simulink model "real_LAB3_SS"  (R2025b)
settings: Solver=ode3  StartTime=0.0  StopTime=10  FixedStep=0.001  RelTol=1e-3
values from neighbouring files (symbols this model uses):
  deltac = 1/sqrt(2)    [real_LAB3.m]    (also in sim_LAB3.m)
  K = lqr(sysG,Q,R)    [diScorta.m]    (also in real_LAB3.m; sim_LAB3.m = place(A, B,lamb))
  Nu = N(5)    [diScorta.m]    (also in real_LAB3.m; sim_LAB3.m)
  Nx = N(1:4)    [diScorta.m]    (also in real_LAB3.m; sim_LAB3.m)
  step_amplitude = 50    [diScorta.m]    (also in real_LAB3.m)
  t0 = 0.2    [diScorta.m]    (also in real_LAB3.m; real_estimation.m)
  t1 = 0.7    [diScorta.m]    (also in real_LAB3.m; real_estimation.m)
  Ts = 0.001    [diScorta.m]    (also in real_LAB3.m; real_estimation.m; sim_LAB3.m)
  wc = 2*pi*50    (= 314.159265359)    [real_LAB3.m]    (also in sim_LAB3.m)
undefined symbols (not defined in the file or in its folder): degs2rpm, DiscIntNeverNeededParam, National_Instruments, PCI, rpm2rads, sens
libraries: sldrtlib x3, simulink x1
settings Model: SimulationMode=external  ExtModeTrigDuration=100001  Creator=delpratogi  LastModifiedBy=ester
settings DataIOCC: ReturnWorkspaceOutputs=off
settings HardwareCC: ProdBitPerLong=64.0  ProdHWDeviceType=Intel->x86-64 (Linux 64)
settings RTWCC: SystemTargetFile=sldrt.tlc  TemplateMakefile=sldrt.tmf  RTWCompilerOptimization=on  Description=Simulink Desktop Real-Time
settings CodeAppCC: MaxIdLength=95.0
settings SimulinkDesktopRealTimeCC: ExtModeTransport=0.0  ExtModeStaticAllocSize=1000000.0  TargetLibSuffix=_sldrt.a  TargetPreCompLibLocation=C:\Program Files\MATLAB\R2025b\toolbox\sldrt\lib\win64  MultiwordLength=2048.0  DynamicStringBufferSize=256.0  ParMdlRefBuildCompliant=on  PreserveMATLABNamespacesInGeneratedCode=on  SubcomponentCodeInterfacePackaging=Reusable function

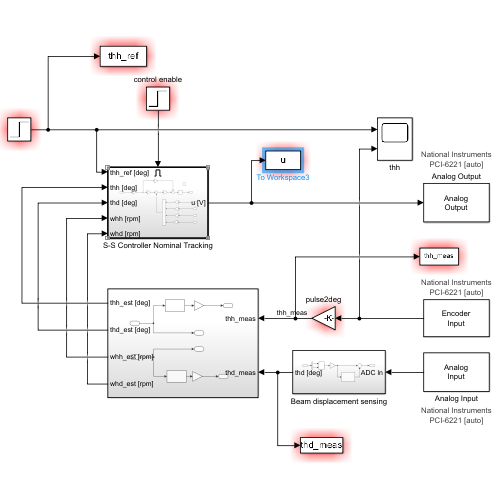
[thumbnail: Simulink's stored preview of the top-level diagram]
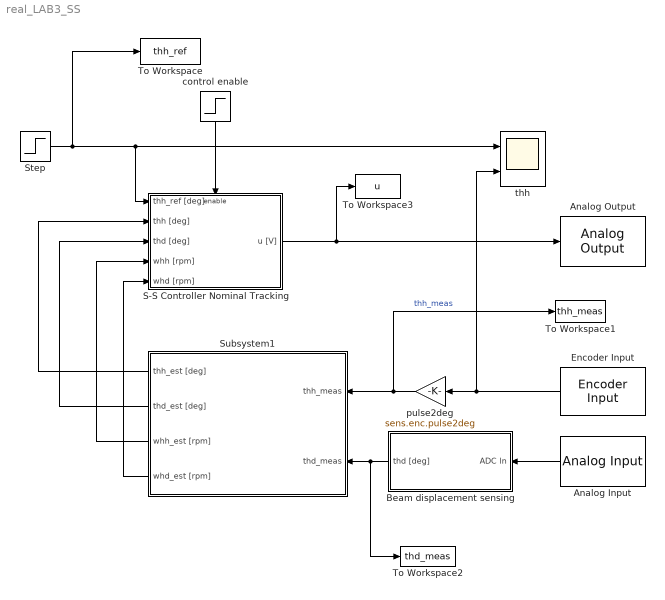
== system real_LAB3_SS ==
  Analog Input : sldrtlib/Analog Input  SampleTime=0.001  MaxMissedTicks=10  ShowMissedTicks=off  YieldWhenWaiting=off  DrvName=National_Instruments/PCI-6221  DrvAddress=4294967295  DrvOptions=[0 0 0 2 0]  Channels=[3,2]  RangeMode=1  VoltRange=2  DataType=1
      settings: AttributesFormatString=National Instruments\nPCI-6221 [auto]
  Analog Output : sldrtlib/Analog Output  SampleTime=0.001  MaxMissedTicks=10  ShowMissedTicks=off  YieldWhenWaiting=off  DrvName=National_Instruments/PCI-6221  DrvAddress=4294967295  DrvOptions=[0 0 0 2 0]  Channels=1  RangeMode=1  VoltRange=1  InitialValue=0  FinalValue=0
      settings: AttributesFormatString=National Instruments\nPCI-6221 [auto]
  Beam displacement sensing : Subsystem
  Encoder Input : sldrtlib/Encoder Input  SampleTime=0.001  MaxMissedTicks=10  ShowMissedTicks=off  YieldWhenWaiting=off  DrvName=National_Instruments/PCI-6221  DrvAddress=4294967295  DrvOptions=[0 0 0 2 0]  Channels=1  QuadMode=3  IndexPulse=1  InputFilter=Inf  DataType=1
      settings: AttributesFormatString=National Instruments\nPCI-6221 [auto]
  S-S Controller Nominal Tracking : Subsystem
  Step : Step  After=step_amplitude  SampleTime=Ts
  Subsystem1 : Subsystem
  To Workspace : ToWorkspace  VariableName=thh_ref  SaveFormat=Structure With Time  SampleTime=Ts
  To Workspace1 : ToWorkspace  VariableName=thh_meas  SaveFormat=Structure With Time  SampleTime=Ts
  To Workspace2 : ToWorkspace  VariableName=thd_meas  SaveFormat=Structure With Time  SampleTime=Ts
  To Workspace3 : ToWorkspace  VariableName=u  SaveFormat=Structure With Time  SampleTime=Ts
  control enable : Step  Time=t1  SampleTime=0
  pulse2deg : Gain  Gain=sens.enc.pulse2deg
  thh : Scope  NumInputPorts=2
      settings: ActiveDisplayYMinimum=-6.2503462089638822  ActiveDisplayYMaximum=56.250038467662655
  wires:
  Analog Input/1 -> Beam displacement sensing/1(ADC ln)
  Subsystem1/2(thd_est [deg]) -> S-S Controller Nominal Tracking/3(thd [deg])
  Step/1 -> To Workspace/1, S-S Controller Nominal Tracking/1(thh_ref [deg]), thh/1
  Subsystem1/3(whh_est [rpm]) -> S-S Controller Nominal Tracking/4(whh [rpm])
  S-S Controller Nominal Tracking/1(u [V]) -> To Workspace3/1, Analog Output/1
  Encoder Input/1 -> thh/2, pulse2deg/1
  Subsystem1/1(thh_est [deg]) -> S-S Controller Nominal Tracking/2(thh [deg])
  Subsystem1/4(whd_est [rpm]) -> S-S Controller Nominal Tracking/5(whd [rpm])
  pulse2deg/1 -> To Workspace1/1, Subsystem1/1(thh_meas)  "thh_meas"
  Beam displacement sensing/1(thd [deg]) -> To Workspace2/1, Subsystem1/2(thd_meas)
  control enable/1 -> S-S Controller Nominal Tracking/Enable

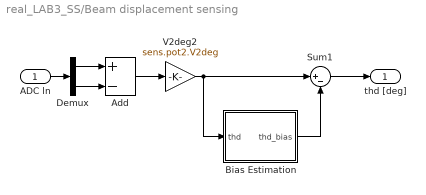
== system real_LAB3_SS/Beam displacement sensing ==
  ADC ln : Inport
  Add : Sum  Inputs=+-
  Bias Estimation : Subsystem
  Demux : Demux  Outputs=2
  Sum1 : Sum  Inputs=|+-
  V2deg2 : Gain  Gain=sens.pot2.V2deg
  thd [deg] : Outport
  wires:
  V2deg2/1 -> Sum1/1, Bias Estimation/1(thd)
  Sum1/1 -> thd [deg]/1
  Bias Estimation/1(thd_bias) -> Sum1/2
  Add/1 -> V2deg2/1
  Demux/1 -> Add/1
  ADC ln/1 -> Demux/1
  Demux/2 -> Add/2

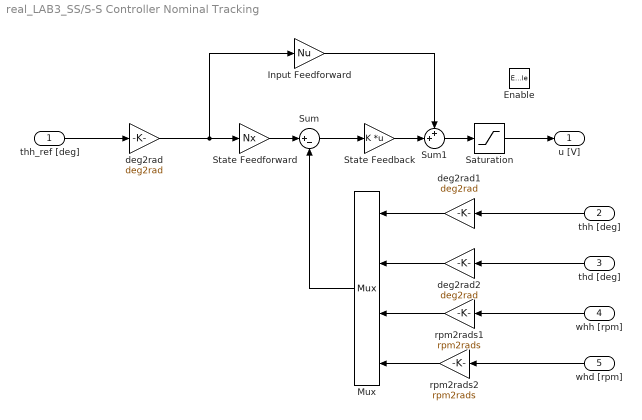
== system real_LAB3_SS/S-S Controller Nominal Tracking ==
  thh_ref [deg] : Inport
  thh [deg] : Inport  Port=2
  thd [deg] : Inport  Port=3
  whh [rpm] : Inport  Port=4
  whd [rpm] : Inport  Port=5
  Enable : EnablePort
  Input Feedforward : Gain  Gain=Nu
  Mux : Mux
  Saturation : Saturate  UpperLimit=10  LowerLimit=-10  ZeroCross=off
  State Feedback : Gain  Gain=K  Multiplication=Matrix(K*u)
  State Feedforward : Gain  Gain=Nx
  Sum : Sum  Inputs=|+-
  Sum1 : Sum  Inputs=++|
  deg2rad : Gain  Gain=deg2rad
  deg2rad1 : Gain  Gain=deg2rad
  deg2rad2 : Gain  Gain=deg2rad
  rpm2rads1 : Gain  Gain=rpm2rads
  rpm2rads2 : Gain  Gain=rpm2rads
  u [V] : Outport
  wires:
  State Feedback/1 -> Sum1/2
  Sum1/1 -> Saturation/1
  Input Feedforward/1 -> Sum1/1
  Sum/1 -> State Feedback/1
  Mux/1 -> Sum/2
  deg2rad/1 -> Input Feedforward/1, State Feedforward/1
  State Feedforward/1 -> Sum/1
  thh_ref [deg]/1 -> deg2rad/1
  Saturation/1 -> u [V]/1
  thh [deg]/1 -> deg2rad1/1
  whh [rpm]/1 -> rpm2rads1/1
  thd [deg]/1 -> deg2rad2/1
  whd [rpm]/1 -> rpm2rads2/1
  deg2rad1/1 -> Mux/1
  rpm2rads2/1 -> Mux/4
  deg2rad2/1 -> Mux/2
  rpm2rads1/1 -> Mux/3

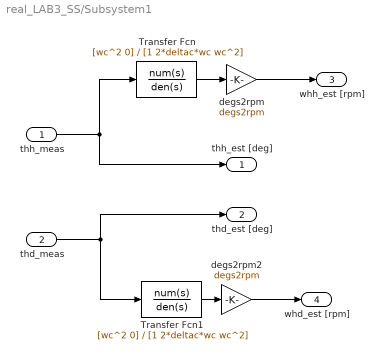
== system real_LAB3_SS/Subsystem1 ==
  thh_meas : Inport
  thd_meas : Inport  Port=2
  Transfer Fcn : TransferFcn  Numerator=[wc^2 0]  Denominator=[1 2*deltac*wc wc^2]
  Transfer Fcn1 : TransferFcn  Numerator=[wc^2 0]  Denominator=[1 2*deltac*wc wc^2]
  degs2rpm : Gain  Gain=degs2rpm
  degs2rpm2 : Gain  Gain=degs2rpm
  thh_est [deg] : Outport
  thd_est [deg] : Outport  Port=2
  whh_est [rpm] : Outport  Port=3
  whd_est [rpm] : Outport  Port=4
  wires:
  thd_meas/1 -> thd_est [deg]/1, Transfer Fcn1/1
  thh_meas/1 -> thh_est [deg]/1, Transfer Fcn/1
  Transfer Fcn/1 -> degs2rpm/1
  degs2rpm2/1 -> whd_est [rpm]/1
  degs2rpm/1 -> whh_est [rpm]/1
  Transfer Fcn1/1 -> degs2rpm2/1

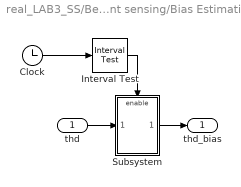
== system real_LAB3_SS/Beam displacement sensing/Bias Estimation ==
  thd : Inport
  Clock : Clock
  Interval Test : simulink/Logic and Bit Operations/Interval Test  IntervalClosedRight=on  uplimit=t1  IntervalClosedLeft=on  lowlimit=t0  OutDataTypeStr=boolean
  Subsystem : Subsystem
  thd_bias : Outport
  wires:
  Interval Test/1 -> Subsystem/Enable
  thd/1 -> Subsystem/1(In1)
  Subsystem/1(Out1) -> thd_bias/1
  Clock/1 -> Interval Test/1

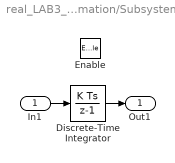
== system real_LAB3_SS/Beam displacement sensing/Bias Estimation/Subsystem ==
  In1 : Inport
  Enable : EnablePort
  Discrete-Time Integrator : DiscreteIntegrator  gainval=1/0.5  SampleTime=Ts  ICPrevOutput=DiscIntNeverNeededParam  ICPrevScaledInput=DiscIntNeverNeededParam
  Out1 : Outport
  wires:
  In1/1 -> Discrete-Time Integrator/1
  Discrete-Time Integrator/1 -> Out1/1
